simulink model "ev_supervisory_control_test"  (R2013a)
settings: Solver=ode3  StartTime=0  StopTime=10000  FixedStep=1  RelTol=1e-3
libraries: simulink x3, CampusEnergyModeling x3
settings Model: Creator=sfrank1  LastModifiedBy=sfrank1

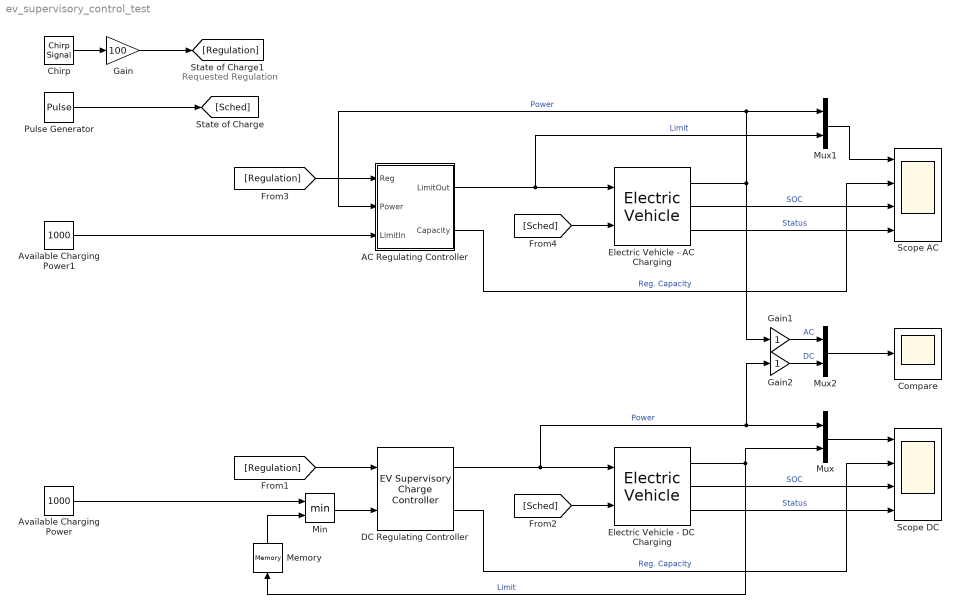
== system ev_supervisory_control_test ==
  note: Requested Regulation
  AC Regulating Controller : Subsystem  mask(DC Charging with Regulation){maxresponse=200, ramp=1}
      mask prompts: maxresponse "Desired +/- regulatory capacity (W)"; ramp "Maximum ramp rate (W/s)"
      mask help: Implements a simple model for an electric vehicle charging station. Accepts connections for the EV state of charge and status as well as an external control signal requesting a regulatory deviation from the current charging setpoint. Outputs a charging power.
      mask Help:
      | Models an electric vehicle charging station
      | 
      | <h2>Description</h2>
      | This block models an idealized electric vehicle (EV) charging station. It is an approximation of how actual EV charging stations operate (to be updated in a later release of the library). The charger uses a preset charging power profile based on the EV battery state of charge (SOC). As the SOC approaches 100%, the charger tapers the charge rate to zero. In addition, the charger monitors the connection status of the EV and sets charging power to zero if the EV is disconnected or has a full battery.
      | 
      | The block has a <b>Control</b> signal which requests regulatory control of the EV charging load as a deviation from the current charging setpoint. This allows the EV charger to participate in demand response or regulation of distributed generation (such as smoothing output from a photovoltaic array). The charger attempts to maintain the active response capability specified in the block mask by operating at less than maximum charging capacity. It can then respond to the control signal within its present charging limits. See Comments for details.
      | 
      | <h2>Input</h2>
      | <dl>
      |   <dt><b>Control</b></dt>
      |     <dd>Signal requesting regulatory control of charging power (&plusmn; deviation from charging setpoint) (W)</dd>
      |   <dt><b>SOC</b></dt>
      |     <dd>EV battery current state of charge (fraction); compatible with the <b>SOC</b> output of the <i>EV Battery</i> block</dd>
      |   <dt><b>Status</b></dt>
      |     <dd>EV status:
      |     <ul>
      |       <li>&minus;1 for not present,</li>
      |       <li>0 for present and accepting charge,</li>
      |       <li>1 for present but battery full;</li>
      |     </ul>
      |     compatible with the <b>Status</b> output of the <i>EV Battery</i> block</dd>
      | </dl>
      | 
      | <h2>Output</h2>
      | Output <b>Power</b> is the charger power output (W).
      | 
      | <h2>Parameters</h2>
      | <dl>
      |   <dt><b>Charger rating</b></dt>
      |     <dd>The charger maximum power rating (W)</dd>
      |   <dt><b>Connected EV battery capacity</b></dt>
      |     <dd>The total energy storage capacity of the connected EV battery (Wh)</dd>
      |   <dt><b>Desired +/- regulatory response capability</b></dt>
      |     <dd>The target control response capability (W) for the charger</dd>
      |   <dt><b>Maximum ramp rate</b></dt>
      |     <dd>Maximum charging ramp rate (&plusmn; rate of change in charging power) (W/s)</dd>
      | </dl>
      | 
      | <h2>Comments</h2>
      | Internally, the block sets a maximum charge rate based on the EV battery capacity and current SOC. The charging setpoint is the maximum rate less any requested regulatory response capability. The actual charging power is equal to this setpoint plus the effect of the control signal.
      | 
      | The ability of the charger to respond to the requested control action is limited by four factors:
      | <ol>
      |   <li>The output power cannot exceed the specified charger power rating.</li>
      |   <li>The output power cannot exceed the maximum charge rate defined by the battery charging profile.</li>
      |   <li>The output power cannot be less than zero. (The battery cannot be discharged to the grid.)</li>
      |   <li>The output power cannot change at a rate greater than the specified maximum ramp rate.</li>
      | </ol>
      | 
      | <i>Example:</i> If, given the current battery SOC, the charging profile for the EV battery specifies 5000 W and the requested regulatory response capability is &plusmn;1000 W, then the EV charger will charge at a setpoint of 4000 W &plusmn; the requested control action, within the limits of the charger. If the requested control action is &minus;500 W, then the EV charger will reduce output to 4000 &minus; 500 = 3500 W.
  Available Charging Power : Constant  Value=1000
  Available Charging Power1 : Constant  Value=1000
  Chirp : simulink/Sources/Chirp Signal  f1=1/3600  T=10e3  f2=1/360
  Compare : Scope
      settings: ShowLegends=on  TimeRange=10000  YMin=0  YMax=900  SaveName=ScopeData2
  DC Regulating Controller : CampusEnergyModeling/Electric Vehicles/EV Supervisory Charge Controller  maxresponse=200  ramp=1
  Electric Vehicle - AC Charging : CampusEnergyModeling/Electric Vehicles/Electric Vehicle  ctype=AC  rating=1000  chargerEff=0.96  profile=off  profileSOC=[0.00 0.10 0.20 0.80 0.99 1.00]  profileRate=[0.10 0.20 1.00 1.00 0.01 0.00]  capacity=1000  initSOC=0.1  battEff=0.98
  Electric Vehicle - DC Charging : CampusEnergyModeling/Electric Vehicles/Electric Vehicle  ctype=DC  rating=6240  chargerEff=0.96  profile=off  profileSOC=[0.00 0.10 0.20 0.80 0.99 1.00]  profileRate=[0.10 0.20 1.00 1.00 0.01 0.00]  capacity=1000  initSOC=0.1  battEff=0.98
  Gain : Gain  Gain=100
  Gain1 : Gain
  Gain2 : Gain
  Memory : Memory
  Min : MinMax  Inputs=2
  Mux : Mux  Inputs=2
  Mux1 : Mux  Inputs=2
  Mux2 : Mux  Inputs=2
  Pulse Generator : DiscretePulseGenerator  PulseType=Time based  Period=10000  PulseWidth=80  PhaseDelay=1000
  Scope AC : Scope  NumInputPorts=4
      settings: ShowLegends=on  TimeRange=10000  YMin=0~0~0~-1  YMax=1000~200~1~0
  Scope DC : Scope  NumInputPorts=4
      settings: ShowLegends=on  TimeRange=10000  YMin=0~0~0~-1  YMax=1000~200~1~0
  wires:
  Electric Vehicle - DC Charging/1 -> Memory/1, Mux/2  "Limit"
  DC Regulating Controller/1 -> Electric Vehicle - DC Charging/1, Gain2/1, Mux/1  "Power"
  Pulse Generator/1 -> [Sched]
  [Sched] -> Electric Vehicle - DC Charging/2
  Available Charging Power/1 -> Min/1
  Chirp/1 -> Gain/1
  Gain/1 -> [Regulation]
  [Regulation] -> DC Regulating Controller/1
  Electric Vehicle - DC Charging/2 -> Scope DC/3  "SOC"
  Electric Vehicle - DC Charging/3 -> Scope DC/4  "Status"
  DC Regulating Controller/2 -> Scope DC/2  "Reg. Capacity"
  Mux/1 -> Scope DC/1
  Memory/1 -> Min/2
  Min/1 -> DC Regulating Controller/2
  AC Regulating Controller/1(LimitOut) -> Mux1/2, Electric Vehicle - AC Charging/1  "Limit"
  [Sched] -> Electric Vehicle - AC Charging/2
  [Regulation] -> AC Regulating Controller/1(Reg)
  Electric Vehicle - AC Charging/2 -> Scope AC/3  "SOC"
  Electric Vehicle - AC Charging/3 -> Scope AC/4  "Status"
  AC Regulating Controller/2(Capacity) -> Scope AC/2  "Reg. Capacity"
  Mux1/1 -> Scope AC/1
  Electric Vehicle - AC Charging/1 -> Gain1/1, Mux1/1, AC Regulating Controller/2(Power)  "Power"
  Available Charging Power1/1 -> AC Regulating Controller/3(LimitIn)
  Mux2/1 -> Compare/1
  Gain1/1 -> Mux2/1  "AC"
  Gain2/1 -> Mux2/2  "DC"

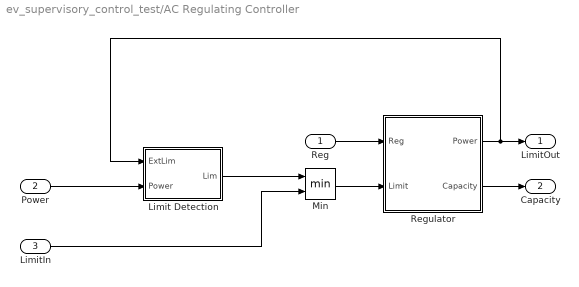
== system ev_supervisory_control_test/AC Regulating Controller ==
  Reg : Inport
  Power : Inport  Port=2
  LimitIn : Inport  Port=3
  Limit Detection : Subsystem
  Min : MinMax  Inputs=2
  Regulator : Subsystem  TreatAsAtomicUnit=on
      settings: RTWFcnNameOpts=Use subsystem name  RTWFileNameOpts=Use function name
  LimitOut : Outport
  Capacity : Outport  Port=2
  wires:
  Reg/1 -> Regulator/1(Reg)
  Regulator/2(Capacity) -> Capacity/1
  Regulator/1(Power) -> Limit Detection/1(ExtLim), LimitOut/1
  Power/1 -> Limit Detection/2(Power)
  Limit Detection/1(Lim) -> Min/1
  Min/1 -> Regulator/2(Limit)
  LimitIn/1 -> Min/2

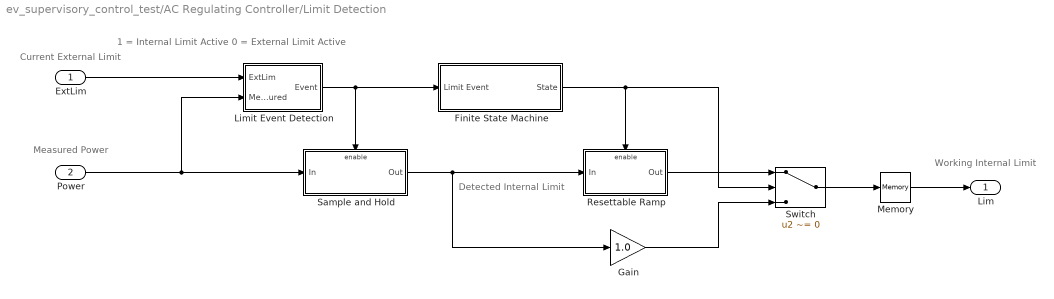
== system ev_supervisory_control_test/AC Regulating Controller/Limit Detection ==
  note: Current External Limit
  note: Measured Power
  note: Working Internal Limit
  note: 1 = Internal Limit Active
      | 0 = External Limit Active
  note: Detected Internal Limit
  ExtLim : Inport
  Power : Inport  Port=2
  Finite State Machine : Subsystem  TreatAsAtomicUnit=on
      settings: RTWFcnNameOpts=Use subsystem name  RTWFileNameOpts=Use function name
  Gain : Gain  Gain=1.0
  Limit Event Detection : Subsystem  TreatAsAtomicUnit=on
      settings: RTWFcnNameOpts=Use subsystem name  RTWFileNameOpts=Use function name
  Memory : Memory
  Resettable Ramp : Subsystem  TreatAsAtomicUnit=on
  Sample and Hold : Subsystem  TreatAsAtomicUnit=on
  Switch : Switch  Criteria=u2 ~= 0
  Lim : Outport
  wires:
  Limit Event Detection/1(Event) -> Finite State Machine/1(Limit Event), Sample and Hold/Enable
  Finite State Machine/1(State) -> Switch/2, Resettable Ramp/Enable
  Resettable Ramp/1(Out) -> Switch/1
  Sample and Hold/1(Out) -> Resettable Ramp/1(In), Gain/1
  Gain/1 -> Switch/3
  Power/1 -> Sample and Hold/1(In), Limit Event Detection/2(Measured)
  Switch/1 -> Memory/1
  ExtLim/1 -> Limit Event Detection/1(ExtLim)
  Memory/1 -> Lim/1

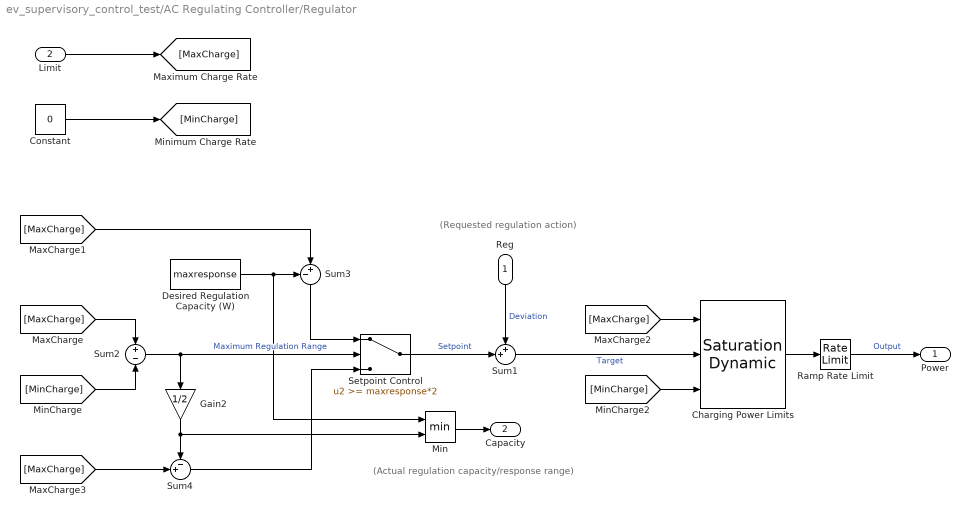
== system ev_supervisory_control_test/AC Regulating Controller/Regulator ==
  note: (Requested regulation action)
  note: (Actual regulation capacity/response range)
  Reg : Inport
  Limit : Inport  Port=2
  Charging Power Limits : simulink/Discontinuities/Saturation Dynamic  OutMin=[]  OutMax=[]  OutDataTypeStr=Inherit: Same as second input  OutDataType=fixdt(1, 16)  OutScaling=2^-10  DoSatur=off
  Constant : Constant  Value=0
  Desired Regulation Capacity (W) : Constant  Value=maxresponse
  Gain2 : Gain  Gain=1/2
  Min : MinMax  Inputs=2
  Ramp Rate Limit : RateLimiter  RisingSlewLimit=ramp  FallingSlewLimit=-ramp  SampleTimeMode=inherited
  Setpoint Control : Switch  Threshold=maxresponse*2
  Sum1 : Sum  Inputs=++|
  Sum2 : Sum  Inputs=+-
  Sum3 : Sum  Inputs=-+|
  Sum4 : Sum  Inputs=-+|
  Power : Outport
  Capacity : Outport  Port=2
  wires:
  Min/1 -> Capacity/1
  Limit/1 -> [MaxCharge]
  Desired Regulation Capacity (W)/1 -> Sum3/1, Min/1
  [MaxCharge] -> Sum3/2
  Sum4/1 -> Setpoint Control/3
  Gain2/1 -> Sum4/1, Min/2
  [MaxCharge] -> Sum4/2
  Sum3/1 -> Setpoint Control/1
  Setpoint Control/1 -> Sum1/2  "Setpoint"
  [MinCharge] -> Sum2/2
  [MaxCharge] -> Sum2/1
  Sum2/1 -> Setpoint Control/2, Gain2/1  "Maximum Regulation Range"
  [MinCharge] -> Charging Power Limits/3
  [MaxCharge] -> Charging Power Limits/1
  Reg/1 -> Sum1/1  "Deviation"
  Constant/1 -> [MinCharge]
  Charging Power Limits/1 -> Ramp Rate Limit/1
  Ramp Rate Limit/1 -> Power/1  "Output"
  Sum1/1 -> Charging Power Limits/2  "Target"

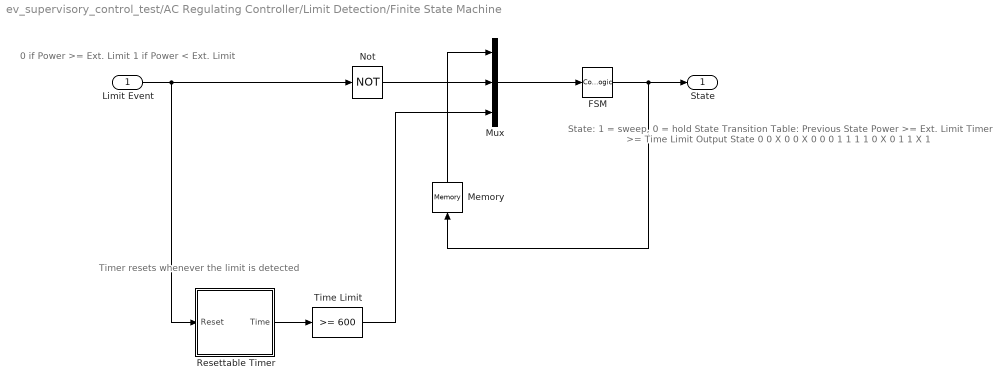
== system ev_supervisory_control_test/AC Regulating Controller/Limit Detection/Finite State Machine ==
  note: Timer resets whenever the limit is detected
  note: 0 if Power >= Ext. Limit
      | 1 if Power < Ext. Limit
  note: State: 1 = sweep, 0 = hold
      |
      | State Transition Table:
      |
      | Previous State	Power >= Ext. Limit	Timer  >= Time Limit		Output State
      | 0				0					X						0
      | 0				X					0						0
      | 0				1					1						1
      | 1				0					X						0
      | 1				1					X						1
  Limit Event : Inport
  FSM : CombinatorialLogic  TruthTable=[0; 0; 0; 1; 0; 0; 1; 1]
  Memory : Memory  X0=1
  Mux : Mux  Inputs=3
  Not : Logic  Operator=NOT  IconShape=distinctive  AllPortsSameDT=off  OutDataTypeStr=boolean
  Resettable Timer : Subsystem  TreatAsAtomicUnit=on
  Time Limit : simulink/Logic and Bit Operations/Compare To Constant  relop=>=  const=600  OutDataTypeStr=boolean
  State : Outport
  wires:
  FSM/1 -> Memory/1, State/1
  Limit Event/1 -> Resettable Timer/1(Reset), Not/1
  Not/1 -> Mux/2
  Mux/1 -> FSM/1
  Time Limit/1 -> Mux/3
  Memory/1 -> Mux/1
  Resettable Timer/1(Time) -> Time Limit/1

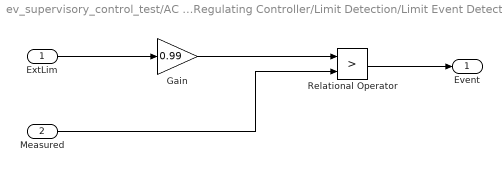
== system ev_supervisory_control_test/AC Regulating Controller/Limit Detection/Limit Event Detection ==
  ExtLim : Inport
  Measured : Inport  Port=2
  Gain : Gain  Gain=0.99
  Relational Operator : RelationalOperator  Operator=>  OutDataTypeStr=boolean
  Event : Outport
  wires:
  Gain/1 -> Relational Operator/1
  ExtLim/1 -> Gain/1
  Relational Operator/1 -> Event/1
  Measured/1 -> Relational Operator/2

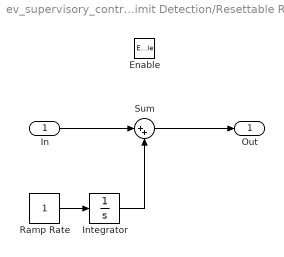
== system ev_supervisory_control_test/AC Regulating Controller/Limit Detection/Resettable Ramp ==
  In : Inport
  Enable : EnablePort  StatesWhenEnabling=reset
  Integrator : Integrator
  Ramp Rate : Constant
  Sum : Sum  Inputs=|++
  Out : Outport
  wires:
  In/1 -> Sum/1
  Sum/1 -> Out/1
  Ramp Rate/1 -> Integrator/1
  Integrator/1 -> Sum/2

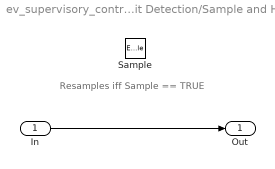
== system ev_supervisory_control_test/AC Regulating Controller/Limit Detection/Sample and Hold ==
  note: Resamples iff Sample == TRUE
  In : Inport
  Sample : EnablePort
  Out : Outport
  wires:
  In/1 -> Out/1

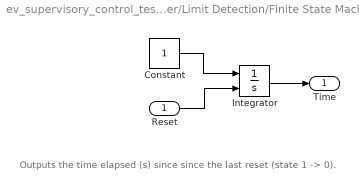
== system ev_supervisory_control_test/AC Regulating Controller/Limit Detection/Finite State Machine/Resettable Timer ==
  note: Outputs the time elapsed (s) since
      | since the last reset (state 1 -> 0).
  Reset : Inport
  Constant : Constant
  Integrator : Integrator  ExternalReset=level
  Time : Outport
  wires:
  Constant/1 -> Integrator/1
  Integrator/1 -> Time/1
  Reset/1 -> Integrator/2
